simulink model "task_3_simm"  (R2023a)
settings: Solver=VariableStepAuto  StartTime=0.0  StopTime=10.0  RelTol=1e-3
undefined symbols (not defined in the file): A, B, C, D, K, L, x0, xh0
settings Model: Creator=user  LastModifiedBy=user

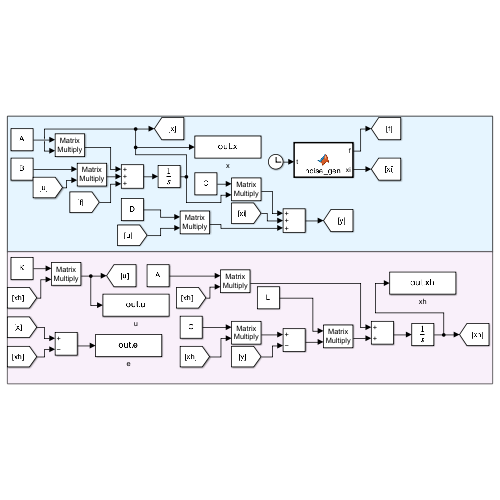
[thumbnail: Simulink's stored preview of the top-level diagram]
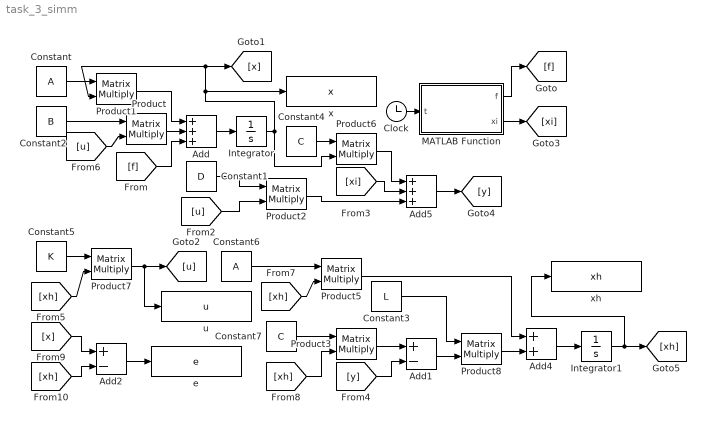
== system task_3_simm ==
  Add : Sum  Inputs=+++
  Add1 : Sum  Inputs=+-
  Add2 : Sum  Inputs=+-
  Add4 : Sum
  Add5 : Sum  Inputs=+++
  Clock : Clock
  Constant : Constant  Value=A  VectorParams1D=off
  Constant1 : Constant  Value=D  VectorParams1D=off
  Constant2 : Constant  Value=B  VectorParams1D=off
  Constant3 : Constant  Value=L  VectorParams1D=off
  Constant4 : Constant  Value=C  VectorParams1D=off
  Constant5 : Constant  Value=K  VectorParams1D=off
  Constant6 : Constant  Value=A  VectorParams1D=off
  Constant7 : Constant  Value=C  VectorParams1D=off
  Integrator : Integrator  InitialCondition=x0
  Integrator1 : Integrator  InitialCondition=xh0
  MATLAB Function : MATLAB Function  TreatAsAtomicUnit=on
  Product{,1..3,5..8} (8 alike) : Product  Multiplication=Matrix(*)
  e : ToWorkspace  VariableName=e  SaveFormat=Timeseries  SampleTime=-1
  u : ToWorkspace  VariableName=u  SaveFormat=Timeseries  SampleTime=-1
  x : ToWorkspace  VariableName=x  SaveFormat=Timeseries  SampleTime=-1
  xh : ToWorkspace  VariableName=xh  SaveFormat=Timeseries  SampleTime=-1
  wires:
  Clock/1 -> MATLAB Function/1(t)
  Constant/1 -> Product1/1
  Product1/1 -> Add/1
  Add/1 -> Integrator/1
  Constant2/1 -> Product/1
  Product/1 -> Add/2
  Integrator/1 -> Product1/2, [x], x/1, Product6/2
  MATLAB Function/1(f) -> [f]
  [f] -> Add/3
  Constant4/1 -> Product6/1
  Constant1/1 -> Product2/1
  MATLAB Function/2(xi) -> [xi]
  [xi] -> Add5/2
  Product6/1 -> Add5/1
  Product2/1 -> Add5/3
  Add5/1 -> [y]
  Constant5/1 -> Product7/1
  [xh] -> Product7/2
  Product7/1 -> [u], u/1
  [u] -> Product/2
  Integrator1/1 -> [xh], xh/1
  Constant7/1 -> Product3/1
  [xh] -> Product3/2
  Product3/1 -> Add1/1
  [y] -> Add1/2
  Add1/1 -> Product8/2
  Constant3/1 -> Product8/1
  Constant6/1 -> Product5/1
  [xh] -> Product5/2
  Product8/1 -> Add4/2
  Product5/1 -> Add4/1
  Add4/1 -> Integrator1/1
  [x] -> Add2/1
  [xh] -> Add2/2
  Add2/1 -> e/1
  [u] -> Product2/2

== matlab function task_3_simm/MATLAB Function ==
  data: t input; f output; xi output
function [f, xi] = noise_gen(t)
    f_amp = [0.5; 0.3; 0.4; 0.2];
    xi_amp = [0.1; 0.15];
    
    f = f_amp .* randn(4,1);
    xi = xi_amp .* randn(2,1);
end
